simulink model "GearIntegration"  (R2021b)
settings: Solver=VariableStepAuto  StartTime=0.0  StopTime=inf  RelTol=1e-3
settings Model: Creator=david  LastModifiedBy=david

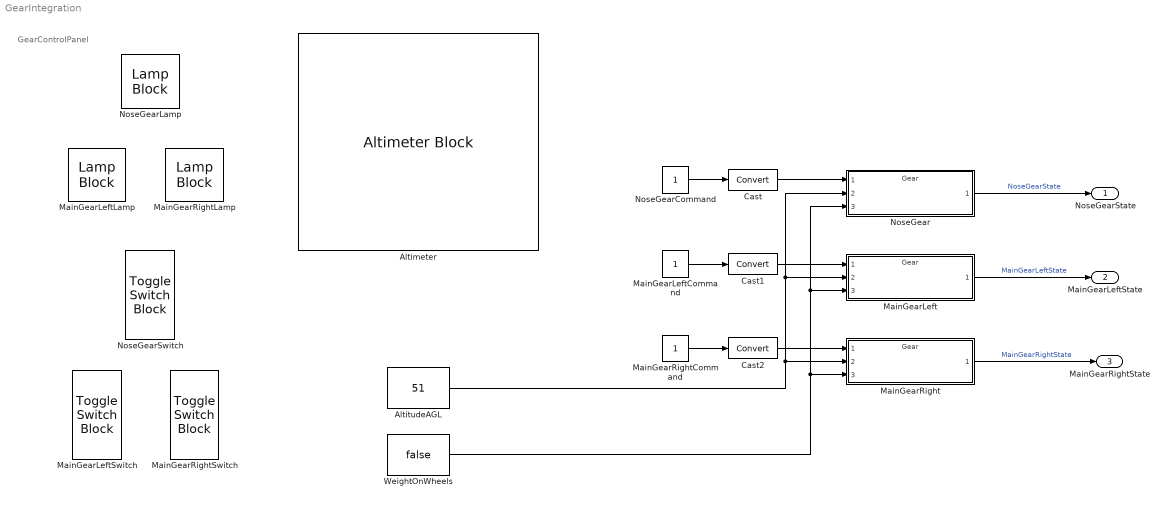
== system GearIntegration ==
  note: GearControlPanel
  Altimeter : AltimeterBlock
  AltitudeAGL : Constant  Value=51
  Cast : DataTypeConversion
  Cast1 : DataTypeConversion
  Cast2 : DataTypeConversion
  MainGearLeft : ModelReference  ModelNameDialog=Gear  SimulationMode=Normal  ModelReferenceVersion=1.18
  MainGearLeftCommand : Constant  OutDataTypeStr=int32
  MainGearLeftLamp : LampBlock  LabelPosition=Hide
  MainGearLeftSwitch : ToggleSwitchBlock
      settings: Values={{'down', 'up'}, [1 0]}
  MainGearRight : ModelReference  ModelNameDialog=Gear  SimulationMode=Normal  ModelReferenceVersion=1.18
  MainGearRightCommand : Constant  OutDataTypeStr=int32
  MainGearRightLamp : LampBlock  LabelPosition=Hide
  MainGearRightSwitch : ToggleSwitchBlock
      settings: Values={{'down', 'up'}, [1 0]}
  NoseGear : ModelReference  ModelNameDialog=Gear  SimulationMode=Normal  ModelReferenceVersion=1.18
  NoseGearCommand : Constant  OutDataTypeStr=int32
  NoseGearLamp : LampBlock  LabelPosition=Hide
  NoseGearSwitch : ToggleSwitchBlock
      settings: Values={{'down', 'up'}, [1 0]}
  WeightOnWheels : Constant  Value=false
  NoseGearState : Outport  OutDataTypeStr=Enum: GearStateEnum
  MainGearLeftState : Outport  Port=2  OutDataTypeStr=Enum: GearStateEnum
  MainGearRightState : Outport  Port=3  OutDataTypeStr=Enum: GearStateEnum
  wires:
  AltitudeAGL/1 -> MainGearLeft/2, NoseGear/2, MainGearRight/2
  NoseGearCommand/1 -> Cast/1
  MainGearLeftCommand/1 -> Cast1/1
  MainGearRightCommand/1 -> Cast2/1
  NoseGear/1 -> NoseGearState/1  "NoseGearState"
  MainGearLeft/1 -> MainGearLeftState/1  "MainGearLeftState"
  MainGearRight/1 -> MainGearRightState/1  "MainGearRightState"
  Cast/1 -> NoseGear/1
  Cast1/1 -> MainGearLeft/1
  Cast2/1 -> MainGearRight/1
  WeightOnWheels/1 -> MainGearRight/3, MainGearLeft/3, NoseGear/3
